simulink model "gm_robot_fis"  (R2023a)
settings: Solver=FixedStepDiscrete  StartTime=0.0  StopTime=10.0  RelTol=1e-3
model workspace (MAT data in the model file):
  x = 1
  y = [100 100 100 100 100 100 100 100 100 100 100 100 ... (256 elements, 256x1)]
libraries: hdlmdlgenlib x75
(part 3 of 3)

== system gm_robot_fis/MinMax Running Resettable4/Subsystem ==
  note: Reset
  note: Xnew
  note: Xold
  u1 : Inport  OutDataTypeStr=uint8  PortDimensions=1  SampleTime=0.2
  R1 : Inport  Port=2  OutDataTypeStr=uint8  PortDimensions=1  SampleTime=0.2
  FixPt Data Type Duplicate2 : DataTypeDuplicate  DisableCoverage=on  NumInputPorts=4
  Initial Condition : Constant  Value=0  OutDataTypeStr=uint8  SampleTime=0.2
  Memory_controlled : Subsystem
  Reset : Switch  Criteria=u2 ~= 0  Threshold=double(0)  OutDataTypeStr=uint8  SampleTime=0.2  SaturateOnIntegerOverflow=off  InputSameDT=off
  delayMatch : Delay  DelayLength=double(1)  InitialCondition=0  SampleTime=0.2
  delayMatch1 : Delay  DelayLength=double(1)  InitialCondition=0  SampleTime=0.2
  delayMatch2 : Delay  DelayLength=double(1)  InitialCondition=0  SampleTime=0.2
  stateControl : Constant  OutDataTypeStr=boolean  SampleTime=0.2
  y1 : Outport  SampleTime=0.2
  x : Outport  Port=2  SampleTime=0.2
  wires:
  delayMatch/1 -> Reset/1
  Memory_controlled/1(out0) -> FixPt Data Type Duplicate2/1, x/1
  Reset/1 -> Memory_controlled/1(in0), FixPt Data Type Duplicate2/2, y1/1
  delayMatch1/1 -> Memory_controlled/Enable
  u1/1 -> Reset/3, FixPt Data Type Duplicate2/4
  R1/1 -> Reset/2
  delayMatch2/1 -> FixPt Data Type Duplicate2/3
  stateControl/1 -> delayMatch1/1
  Initial Condition/1 -> delayMatch2/1, delayMatch/1

== system gm_robot_fis/MinMax Running Resettable5/Subsystem ==
  note: Reset
  note: Xnew
  note: Xold
  u1 : Inport  OutDataTypeStr=uint8  PortDimensions=1  SampleTime=0.2
  R1 : Inport  Port=2  OutDataTypeStr=uint8  PortDimensions=1  SampleTime=0.2
  FixPt Data Type Duplicate2 : DataTypeDuplicate  DisableCoverage=on  NumInputPorts=4
  Initial Condition : Constant  Value=0  OutDataTypeStr=uint8  SampleTime=0.2
  Memory_controlled : Subsystem
  Reset : Switch  Criteria=u2 ~= 0  Threshold=double(0)  OutDataTypeStr=uint8  SampleTime=0.2  SaturateOnIntegerOverflow=off  InputSameDT=off
  delayMatch : Delay  DelayLength=double(1)  InitialCondition=0  SampleTime=0.2
  delayMatch1 : Delay  DelayLength=double(1)  InitialCondition=0  SampleTime=0.2
  delayMatch2 : Delay  DelayLength=double(1)  InitialCondition=0  SampleTime=0.2
  stateControl : Constant  OutDataTypeStr=boolean  SampleTime=0.2
  y1 : Outport  SampleTime=0.2
  x : Outport  Port=2  SampleTime=0.2
  wires:
  delayMatch/1 -> Reset/1
  Memory_controlled/1(out0) -> FixPt Data Type Duplicate2/1, x/1
  Reset/1 -> Memory_controlled/1(in0), FixPt Data Type Duplicate2/2, y1/1
  delayMatch1/1 -> Memory_controlled/Enable
  u1/1 -> Reset/3, FixPt Data Type Duplicate2/4
  R1/1 -> Reset/2
  delayMatch2/1 -> FixPt Data Type Duplicate2/3
  stateControl/1 -> delayMatch1/1
  Initial Condition/1 -> delayMatch2/1, delayMatch/1

== system gm_robot_fis/MinMax Running Resettable6/Subsystem ==
  note: Reset
  note: Xnew
  note: Xold
  u1 : Inport  OutDataTypeStr=uint8  PortDimensions=1  SampleTime=0.2
  R1 : Inport  Port=2  OutDataTypeStr=uint8  PortDimensions=1  SampleTime=0.2
  FixPt Data Type Duplicate2 : DataTypeDuplicate  DisableCoverage=on  NumInputPorts=4
  Initial Condition : Constant  Value=0  OutDataTypeStr=uint8  SampleTime=0.2
  Memory_controlled : Subsystem
  Reset : Switch  Criteria=u2 ~= 0  Threshold=double(0)  OutDataTypeStr=uint8  SampleTime=0.2  SaturateOnIntegerOverflow=off  InputSameDT=off
  delayMatch : Delay  DelayLength=double(1)  InitialCondition=0  SampleTime=0.2
  delayMatch1 : Delay  DelayLength=double(1)  InitialCondition=0  SampleTime=0.2
  delayMatch2 : Delay  DelayLength=double(1)  InitialCondition=0  SampleTime=0.2
  stateControl : Constant  OutDataTypeStr=boolean  SampleTime=0.2
  y1 : Outport  SampleTime=0.2
  x : Outport  Port=2  SampleTime=0.2
  wires:
  delayMatch/1 -> Reset/1
  Memory_controlled/1(out0) -> FixPt Data Type Duplicate2/1, x/1
  Reset/1 -> Memory_controlled/1(in0), FixPt Data Type Duplicate2/2, y1/1
  delayMatch1/1 -> Memory_controlled/Enable
  u1/1 -> Reset/3, FixPt Data Type Duplicate2/4
  R1/1 -> Reset/2
  delayMatch2/1 -> FixPt Data Type Duplicate2/3
  stateControl/1 -> delayMatch1/1
  Initial Condition/1 -> delayMatch2/1, delayMatch/1

== system gm_robot_fis/MinMax Running Resettable7/Subsystem ==
  note: Reset
  note: Xnew
  note: Xold
  u1 : Inport  OutDataTypeStr=uint8  PortDimensions=1  SampleTime=0.2
  R1 : Inport  Port=2  OutDataTypeStr=uint8  PortDimensions=1  SampleTime=0.2
  FixPt Data Type Duplicate2 : DataTypeDuplicate  DisableCoverage=on  NumInputPorts=4
  Initial Condition : Constant  Value=0  OutDataTypeStr=uint8  SampleTime=0.2
  Memory_controlled : Subsystem
  Reset : Switch  Criteria=u2 ~= 0  Threshold=double(0)  OutDataTypeStr=uint8  SampleTime=0.2  SaturateOnIntegerOverflow=off  InputSameDT=off
  delayMatch : Delay  DelayLength=double(1)  InitialCondition=0  SampleTime=0.2
  delayMatch1 : Delay  DelayLength=double(1)  InitialCondition=0  SampleTime=0.2
  delayMatch2 : Delay  DelayLength=double(1)  InitialCondition=0  SampleTime=0.2
  stateControl : Constant  OutDataTypeStr=boolean  SampleTime=0.2
  y1 : Outport  SampleTime=0.2
  x : Outport  Port=2  SampleTime=0.2
  wires:
  delayMatch/1 -> Reset/1
  Memory_controlled/1(out0) -> FixPt Data Type Duplicate2/1, x/1
  Reset/1 -> Memory_controlled/1(in0), FixPt Data Type Duplicate2/2, y1/1
  delayMatch1/1 -> Memory_controlled/Enable
  u1/1 -> Reset/3, FixPt Data Type Duplicate2/4
  R1/1 -> Reset/2
  delayMatch2/1 -> FixPt Data Type Duplicate2/3
  stateControl/1 -> delayMatch1/1
  Initial Condition/1 -> delayMatch2/1, delayMatch/1

== system gm_robot_fis/MinMax Running Resettable8/Subsystem ==
  note: Reset
  note: Xnew
  note: Xold
  u1 : Inport  OutDataTypeStr=uint8  PortDimensions=1  SampleTime=0.2
  R1 : Inport  Port=2  OutDataTypeStr=uint8  PortDimensions=1  SampleTime=0.2
  FixPt Data Type Duplicate2 : DataTypeDuplicate  DisableCoverage=on  NumInputPorts=4
  Initial Condition : Constant  Value=0  OutDataTypeStr=uint8  SampleTime=0.2
  Memory_controlled : Subsystem
  Reset : Switch  Criteria=u2 ~= 0  Threshold=double(0)  OutDataTypeStr=uint8  SampleTime=0.2  SaturateOnIntegerOverflow=off  InputSameDT=off
  delayMatch : Delay  DelayLength=double(1)  InitialCondition=0  SampleTime=0.2
  delayMatch1 : Delay  DelayLength=double(1)  InitialCondition=0  SampleTime=0.2
  delayMatch2 : Delay  DelayLength=double(1)  InitialCondition=0  SampleTime=0.2
  stateControl : Constant  OutDataTypeStr=boolean  SampleTime=0.2
  y1 : Outport  SampleTime=0.2
  x : Outport  Port=2  SampleTime=0.2
  wires:
  delayMatch/1 -> Reset/1
  Memory_controlled/1(out0) -> FixPt Data Type Duplicate2/1, x/1
  Reset/1 -> Memory_controlled/1(in0), FixPt Data Type Duplicate2/2, y1/1
  delayMatch1/1 -> Memory_controlled/Enable
  u1/1 -> Reset/3, FixPt Data Type Duplicate2/4
  R1/1 -> Reset/2
  delayMatch2/1 -> FixPt Data Type Duplicate2/3
  stateControl/1 -> delayMatch1/1
  Initial Condition/1 -> delayMatch2/1, delayMatch/1

== system gm_robot_fis/MinMax Running Resettable9/Subsystem ==
  note: Reset
  note: Xnew
  note: Xold
  u1 : Inport  OutDataTypeStr=uint8  PortDimensions=1  SampleTime=0.2
  R1 : Inport  Port=2  OutDataTypeStr=uint8  PortDimensions=1  SampleTime=0.2
  FixPt Data Type Duplicate2 : DataTypeDuplicate  DisableCoverage=on  NumInputPorts=4
  Initial Condition : Constant  Value=0  OutDataTypeStr=uint8  SampleTime=0.2
  Memory_controlled : Subsystem
  Reset : Switch  Criteria=u2 ~= 0  Threshold=double(0)  OutDataTypeStr=uint8  SampleTime=0.2  SaturateOnIntegerOverflow=off  InputSameDT=off
  delayMatch : Delay  DelayLength=double(1)  InitialCondition=0  SampleTime=0.2
  delayMatch1 : Delay  DelayLength=double(1)  InitialCondition=0  SampleTime=0.2
  delayMatch2 : Delay  DelayLength=double(1)  InitialCondition=0  SampleTime=0.2
  stateControl : Constant  OutDataTypeStr=boolean  SampleTime=0.2
  y1 : Outport  SampleTime=0.2
  x : Outport  Port=2  SampleTime=0.2
  wires:
  delayMatch/1 -> Reset/1
  Memory_controlled/1(out0) -> FixPt Data Type Duplicate2/1, x/1
  Reset/1 -> Memory_controlled/1(in0), FixPt Data Type Duplicate2/2, y1/1
  delayMatch1/1 -> Memory_controlled/Enable
  u1/1 -> Reset/3, FixPt Data Type Duplicate2/4
  R1/1 -> Reset/2
  delayMatch2/1 -> FixPt Data Type Duplicate2/3
  stateControl/1 -> delayMatch1/1
  Initial Condition/1 -> delayMatch2/1, delayMatch/1

== system gm_robot_fis/MinMax Running Resettable/Subsystem/Memory_controlled ==
  in0 : Inport  OutDataTypeStr=uint8  SampleTime=0.2
  stateControl : EnablePort  OutDataTypeStr=boolean
  Memory : UnitDelay  InitialCondition=double(0)  SampleTime=0.2
  out0 : Outport  OutDataTypeStr=uint8  SampleTime=0.2
  wires:
  Memory/1 -> out0/1
  in0/1 -> Memory/1

== system gm_robot_fis/MinMax Running Resettable1/Subsystem/Memory_controlled ==
  in0 : Inport  OutDataTypeStr=uint8  SampleTime=0.2
  stateControl : EnablePort  OutDataTypeStr=boolean
  Memory : UnitDelay  InitialCondition=double(0)  SampleTime=0.2
  out0 : Outport  OutDataTypeStr=uint8  SampleTime=0.2
  wires:
  Memory/1 -> out0/1
  in0/1 -> Memory/1

== system gm_robot_fis/MinMax Running Resettable10/Subsystem/Memory_controlled ==
  in0 : Inport  OutDataTypeStr=uint8  SampleTime=0.2
  stateControl : EnablePort  OutDataTypeStr=boolean
  Memory : UnitDelay  InitialCondition=double(0)  SampleTime=0.2
  out0 : Outport  OutDataTypeStr=uint8  SampleTime=0.2
  wires:
  Memory/1 -> out0/1
  in0/1 -> Memory/1

== system gm_robot_fis/MinMax Running Resettable11/Subsystem/Memory_controlled ==
  in0 : Inport  OutDataTypeStr=uint8  SampleTime=0.2
  stateControl : EnablePort  OutDataTypeStr=boolean
  Memory : UnitDelay  InitialCondition=double(0)  SampleTime=0.2
  out0 : Outport  OutDataTypeStr=uint8  SampleTime=0.2
  wires:
  Memory/1 -> out0/1
  in0/1 -> Memory/1

== system gm_robot_fis/MinMax Running Resettable12/Subsystem/Memory_controlled ==
  in0 : Inport  OutDataTypeStr=uint8  SampleTime=0.2
  stateControl : EnablePort  OutDataTypeStr=boolean
  Memory : UnitDelay  InitialCondition=double(0)  SampleTime=0.2
  out0 : Outport  OutDataTypeStr=uint8  SampleTime=0.2
  wires:
  Memory/1 -> out0/1
  in0/1 -> Memory/1

== system gm_robot_fis/MinMax Running Resettable13/Subsystem/Memory_controlled ==
  in0 : Inport  OutDataTypeStr=uint8  SampleTime=0.2
  stateControl : EnablePort  OutDataTypeStr=boolean
  Memory : UnitDelay  InitialCondition=double(0)  SampleTime=0.2
  out0 : Outport  OutDataTypeStr=uint8  SampleTime=0.2
  wires:
  Memory/1 -> out0/1
  in0/1 -> Memory/1

== system gm_robot_fis/MinMax Running Resettable14/Subsystem/Memory_controlled ==
  in0 : Inport  OutDataTypeStr=uint8  SampleTime=0.2
  stateControl : EnablePort  OutDataTypeStr=boolean
  Memory : UnitDelay  InitialCondition=double(0)  SampleTime=0.2
  out0 : Outport  OutDataTypeStr=uint8  SampleTime=0.2
  wires:
  Memory/1 -> out0/1
  in0/1 -> Memory/1

== system gm_robot_fis/MinMax Running Resettable15/Subsystem/Memory_controlled ==
  in0 : Inport  OutDataTypeStr=uint8  SampleTime=0.2
  stateControl : EnablePort  OutDataTypeStr=boolean
  Memory : UnitDelay  InitialCondition=double(0)  SampleTime=0.2
  out0 : Outport  OutDataTypeStr=uint8  SampleTime=0.2
  wires:
  Memory/1 -> out0/1
  in0/1 -> Memory/1

== system gm_robot_fis/MinMax Running Resettable16/Subsystem/Memory_controlled ==
  in0 : Inport  OutDataTypeStr=uint8  SampleTime=0.2
  stateControl : EnablePort  OutDataTypeStr=boolean
  Memory : UnitDelay  InitialCondition=double(0)  SampleTime=0.2
  out0 : Outport  OutDataTypeStr=uint8  SampleTime=0.2
  wires:
  Memory/1 -> out0/1
  in0/1 -> Memory/1

== system gm_robot_fis/MinMax Running Resettable17/Subsystem/Memory_controlled ==
  in0 : Inport  OutDataTypeStr=uint8  SampleTime=0.2
  stateControl : EnablePort  OutDataTypeStr=boolean
  Memory : UnitDelay  InitialCondition=double(0)  SampleTime=0.2
  out0 : Outport  OutDataTypeStr=uint8  SampleTime=0.2
  wires:
  Memory/1 -> out0/1
  in0/1 -> Memory/1

== system gm_robot_fis/MinMax Running Resettable18/Subsystem/Memory_controlled ==
  in0 : Inport  OutDataTypeStr=uint8  SampleTime=0.2
  stateControl : EnablePort  OutDataTypeStr=boolean
  Memory : UnitDelay  InitialCondition=double(0)  SampleTime=0.2
  out0 : Outport  OutDataTypeStr=uint8  SampleTime=0.2
  wires:
  Memory/1 -> out0/1
  in0/1 -> Memory/1

== system gm_robot_fis/MinMax Running Resettable19/Subsystem/Memory_controlled ==
  in0 : Inport  OutDataTypeStr=uint8  SampleTime=0.2
  stateControl : EnablePort  OutDataTypeStr=boolean
  Memory : UnitDelay  InitialCondition=double(0)  SampleTime=0.2
  out0 : Outport  OutDataTypeStr=uint8  SampleTime=0.2
  wires:
  Memory/1 -> out0/1
  in0/1 -> Memory/1

== system gm_robot_fis/MinMax Running Resettable20/Subsystem/Memory_controlled ==
  in0 : Inport  OutDataTypeStr=uint8  SampleTime=0.2
  stateControl : EnablePort  OutDataTypeStr=boolean
  Memory : UnitDelay  InitialCondition=double(0)  SampleTime=0.2
  out0 : Outport  OutDataTypeStr=uint8  SampleTime=0.2
  wires:
  Memory/1 -> out0/1
  in0/1 -> Memory/1

== system gm_robot_fis/MinMax Running Resettable21/Subsystem/Memory_controlled ==
  in0 : Inport  OutDataTypeStr=uint8  SampleTime=0.2
  stateControl : EnablePort  OutDataTypeStr=boolean
  Memory : UnitDelay  InitialCondition=double(0)  SampleTime=0.2
  out0 : Outport  OutDataTypeStr=uint8  SampleTime=0.2
  wires:
  Memory/1 -> out0/1
  in0/1 -> Memory/1

== system gm_robot_fis/MinMax Running Resettable22/Subsystem/Memory_controlled ==
  in0 : Inport  OutDataTypeStr=uint8  SampleTime=0.2
  stateControl : EnablePort  OutDataTypeStr=boolean
  Memory : UnitDelay  InitialCondition=double(0)  SampleTime=0.2
  out0 : Outport  OutDataTypeStr=uint8  SampleTime=0.2
  wires:
  Memory/1 -> out0/1
  in0/1 -> Memory/1

== system gm_robot_fis/MinMax Running Resettable23/Subsystem/Memory_controlled ==
  in0 : Inport  OutDataTypeStr=uint8  SampleTime=0.2
  stateControl : EnablePort  OutDataTypeStr=boolean
  Memory : UnitDelay  InitialCondition=double(0)  SampleTime=0.2
  out0 : Outport  OutDataTypeStr=uint8  SampleTime=0.2
  wires:
  Memory/1 -> out0/1
  in0/1 -> Memory/1

== system gm_robot_fis/MinMax Running Resettable24/Subsystem/Memory_controlled ==
  in0 : Inport  OutDataTypeStr=uint8  SampleTime=0.2
  stateControl : EnablePort  OutDataTypeStr=boolean
  Memory : UnitDelay  InitialCondition=double(0)  SampleTime=0.2
  out0 : Outport  OutDataTypeStr=uint8  SampleTime=0.2
  wires:
  Memory/1 -> out0/1
  in0/1 -> Memory/1

== system gm_robot_fis/MinMax Running Resettable25/Subsystem/Memory_controlled ==
  in0 : Inport  OutDataTypeStr=uint8  SampleTime=0.2
  stateControl : EnablePort  OutDataTypeStr=boolean
  Memory : UnitDelay  InitialCondition=double(0)  SampleTime=0.2
  out0 : Outport  OutDataTypeStr=uint8  SampleTime=0.2
  wires:
  Memory/1 -> out0/1
  in0/1 -> Memory/1

== system gm_robot_fis/MinMax Running Resettable3/Subsystem/Memory_controlled ==
  in0 : Inport  OutDataTypeStr=uint8  SampleTime=0.2
  stateControl : EnablePort  OutDataTypeStr=boolean
  Memory : UnitDelay  InitialCondition=double(0)  SampleTime=0.2
  out0 : Outport  OutDataTypeStr=uint8  SampleTime=0.2
  wires:
  Memory/1 -> out0/1
  in0/1 -> Memory/1

== system gm_robot_fis/MinMax Running Resettable4/Subsystem/Memory_controlled ==
  in0 : Inport  OutDataTypeStr=uint8  SampleTime=0.2
  stateControl : EnablePort  OutDataTypeStr=boolean
  Memory : UnitDelay  InitialCondition=double(0)  SampleTime=0.2
  out0 : Outport  OutDataTypeStr=uint8  SampleTime=0.2
  wires:
  Memory/1 -> out0/1
  in0/1 -> Memory/1

== system gm_robot_fis/MinMax Running Resettable5/Subsystem/Memory_controlled ==
  in0 : Inport  OutDataTypeStr=uint8  SampleTime=0.2
  stateControl : EnablePort  OutDataTypeStr=boolean
  Memory : UnitDelay  InitialCondition=double(0)  SampleTime=0.2
  out0 : Outport  OutDataTypeStr=uint8  SampleTime=0.2
  wires:
  Memory/1 -> out0/1
  in0/1 -> Memory/1

== system gm_robot_fis/MinMax Running Resettable6/Subsystem/Memory_controlled ==
  in0 : Inport  OutDataTypeStr=uint8  SampleTime=0.2
  stateControl : EnablePort  OutDataTypeStr=boolean
  Memory : UnitDelay  InitialCondition=double(0)  SampleTime=0.2
  out0 : Outport  OutDataTypeStr=uint8  SampleTime=0.2
  wires:
  Memory/1 -> out0/1
  in0/1 -> Memory/1

== system gm_robot_fis/MinMax Running Resettable7/Subsystem/Memory_controlled ==
  in0 : Inport  OutDataTypeStr=uint8  SampleTime=0.2
  stateControl : EnablePort  OutDataTypeStr=boolean
  Memory : UnitDelay  InitialCondition=double(0)  SampleTime=0.2
  out0 : Outport  OutDataTypeStr=uint8  SampleTime=0.2
  wires:
  Memory/1 -> out0/1
  in0/1 -> Memory/1

== system gm_robot_fis/MinMax Running Resettable8/Subsystem/Memory_controlled ==
  in0 : Inport  OutDataTypeStr=uint8  SampleTime=0.2
  stateControl : EnablePort  OutDataTypeStr=boolean
  Memory : UnitDelay  InitialCondition=double(0)  SampleTime=0.2
  out0 : Outport  OutDataTypeStr=uint8  SampleTime=0.2
  wires:
  Memory/1 -> out0/1
  in0/1 -> Memory/1

== system gm_robot_fis/MinMax Running Resettable9/Subsystem/Memory_controlled ==
  in0 : Inport  OutDataTypeStr=uint8  SampleTime=0.2
  stateControl : EnablePort  OutDataTypeStr=boolean
  Memory : UnitDelay  InitialCondition=double(0)  SampleTime=0.2
  out0 : Outport  OutDataTypeStr=uint8  SampleTime=0.2
  wires:
  Memory/1 -> out0/1
  in0/1 -> Memory/1

== matlab function gm_robot_fis/MATLAB Function/MATLAB Function ==
  data: a input; y output; b input; c input; d input; e input
function y = fcn(a,b,c,d,e)
max = a;
y = uint8(0);
if (b > max)
    max = b;
    y = uint8(1);
end
if (c > max)
    max = c;
    y = uint8(2);
end
if (d > max)
    max = d;
    y = uint8(3);
end
if (e > max)
    y = uint8(4);
end
